simulink model "model2"  (R2015a)
settings: Solver=ode45  StartTime=0.0  StopTime=17  RelTol=1e-3
values from neighbouring files (symbols this model uses):
  den = [1 2*wn*z wn^2]    [logic.m]
  num = [K*wn^2]    [logic.m]
undefined symbols (not defined in the file or in its folder): L, R
settings Model: Creator=Daniel Santos  LastModifiedBy=Daniel Santos

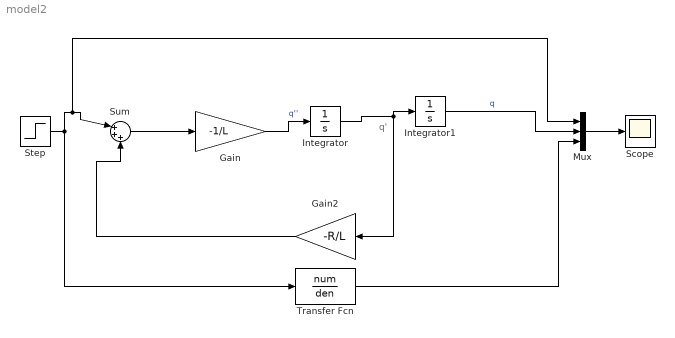
== system model2 ==
  note: q'
  Gain : Gain  Gain=-1/L
  Gain2 : Gain  Gain=-R/L
  Integrator : Integrator
  Integrator1 : Integrator  InitialCondition=0.01
  Mux : Mux  Inputs=3
  Scope : Scope
  Step : Step  Time=0  SampleTime=0
  Sum : Sum  Inputs=|+++
  Transfer Fcn : TransferFcn  Numerator=num  Denominator=den
  wires:
  Gain/1 -> Integrator/1  "q''"
  Integrator/1 -> Gain2/1, Integrator1/1
  Gain2/1 -> Sum/3
  Integrator1/1 -> Mux/2  "q"
  Sum/1 -> Gain/1
  Mux/1 -> Scope/1
  Transfer Fcn/1 -> Mux/3
  Step/1 -> Transfer Fcn/1, Mux/1, Sum/1
